simulink model "Fig261"  (R2014b)
settings: Solver=ode3  StartTime=0.0  StopTime=100  FixedStep=2e-5  RelTol=1e-5
undefined symbols (not defined in the file): gcbh, rcfiltgaincompat
libraries: commfilt2 x2, commrandsrc2 x1, dspstat3 x1
settings Model: Creator=Dennis Silage  LastModifiedBy=Silage
settings DataIOCC: SignalLoggingSaveFormat=ModelDataLogs
settings OptimizationCC: ExpressionDepthLimit=2147483647  InitFltsAndDblsToZero=on
settings DebuggingCC: UnderspecifiedInitializationDetection=Classic  MergeDetectMultiDrivingBlocksExec=none  SolverPrmCheckMsg=none  FcnCallInpInsideContextMsg=UseLocalSettings  StateNameClashWarn=warning
settings GRTTargetCC: CombineOutputUpdateFcns=off  GRTInterface=on

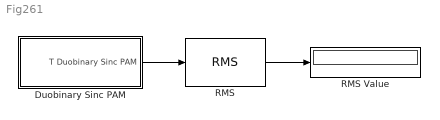
== system Fig261 ==
  Duobinary Sinc PAM : Subsystem
  RMS : dspstat3/RMS  run=on  reset_popup=None  InputProcessing=Inherited (this choice will be removed - see release notes)  directionMode=Each column  dimension=1  treatSBRowAsCol=on
  RMS Value : Display
  wires:
  RMS/1 -> RMS Value/1
  Duobinary Sinc PAM/1(T Duobinary Sinc PAM) -> RMS/1

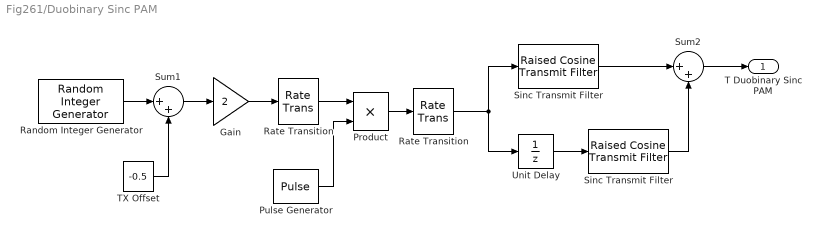
== system Fig261/Duobinary Sinc PAM ==
  " Rate Transition" : RateTransition  OutPortSampleTime=1e-3
  Gain : Gain  Gain=2
  Product : Product  RndMeth=Zero
  Pulse Generator : DiscretePulseGenerator  PulseType=Time based  Period=1e-3  PulseWidth=2
  Random Integer Generator : commrandsrc2/Random Integer Generator  mul=2  seed=randseed  Ts=1e-3  frameBased=off  sampPerFrame=50  orient=off  outDataType=double
  Rate Transition : RateTransition  OutPortSampleTime=2e-5
  Sinc Transmit Filter : commfilt2/Raised Cosine Transmit Filter  filtType=Normal  filtSpan=2*(4)  currentFiltSpan=2*(4)  D=4  R=0  sampMode=Mute  saveAsFlag=0  N=50  framing=Maintain input frame size  InputProcessing=Inherited (this choice will be removed - see release notes)  checkGain=User-specified  filterGain=(5)*rcfiltgaincompat(gcbh)  checkCoeff=off  variableName=rcTxFilt  launchFVT=off  roundingMode=Floor  overflowMode=off
  "Sinc Transmit Filter " : commfilt2/Raised Cosine Transmit Filter  filtType=Normal  filtSpan=2*(4)  currentFiltSpan=2*(4)  D=4  R=0  sampMode=Mute  saveAsFlag=0  N=50  framing=Maintain input frame size  InputProcessing=Inherited (this choice will be removed - see release notes)  checkGain=User-specified  filterGain=(5)*rcfiltgaincompat(gcbh)  checkCoeff=off  variableName=rcTxFilt1  launchFVT=off  roundingMode=Floor  overflowMode=off
  Sum1 : Sum  Inputs=|++
  Sum2 : Sum  Inputs=|++
  TX Offset : Constant  Value=-0.5
  Unit Delay : UnitDelay  SampleTime=-1
  T Duobinary Sinc PAM : Outport
  wires:
  Unit Delay/1 -> "Sinc Transmit Filter "/1
  Sinc Transmit Filter/1 -> Sum2/1
  "Sinc Transmit Filter "/1 -> Sum2/2
  Product/1 -> " Rate Transition"/1
  " Rate Transition"/1 -> Sinc Transmit Filter/1, Unit Delay/1
  Pulse Generator/1 -> Product/2
  Rate Transition/1 -> Product/1
  Gain/1 -> Rate Transition/1
  Random Integer Generator/1 -> Sum1/1
  TX Offset/1 -> Sum1/2
  Sum1/1 -> Gain/1
  Sum2/1 -> T Duobinary Sinc PAM/1
